simulink model "lab7_block"  (R2017b)
settings: Solver=VariableStepAuto  StartTime=0.0  StopTime=10  MaxStep=0.001  RelTol=1e-3
settings Model: Creator=user  LastModifiedBy=HONOR
settings SolverCC: AutoInsertRateTranBlk=on
settings DataIOCC: LimitDataPoints=on  SaveOutput=off  SignalLogging=off  SaveTime=off
settings OptimizationCC: LifeSpan=inf
settings DebuggingCC: AlgebraicLoopMsg=error  SingleTaskRateTransMsg=error  AllowSymbolicDim=off  SFUnexpectedBacktrackingDiag=warning  SFNoUnconditionalDefaultTransitionDiag=warning  SFExecutionAtInitializationDiag=none
settings CodeAppCC: StateflowObjectComments=on
settings GRTTargetCC: TargetLangStandard=C89/C90 (ANSI)  GeneratePreprocessorConditionals=Disable all
settings ConfigComp: CovMetricSettings=dw  CovHtmlReporting=on  CovSaveCumulativeToWorkspaceVar=on  CovSaveSingleToWorkspaceVar=on  CovExternalEMLEnable=off

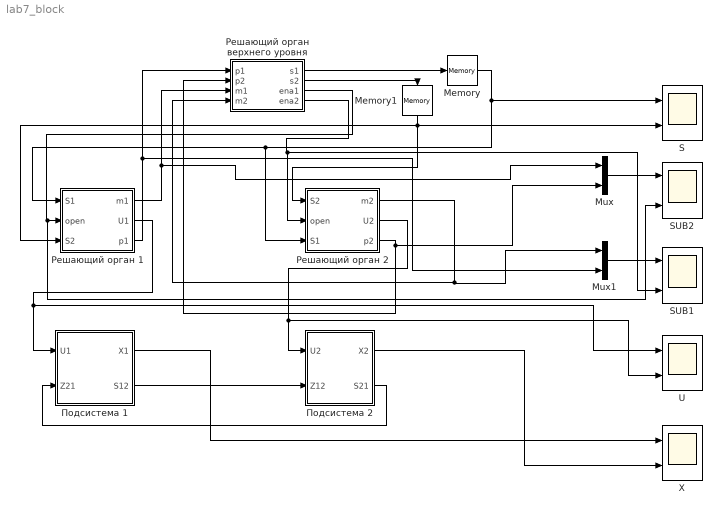
== system lab7_block ==
  Memory : Memory  InitialCondition=0.5
  Memory1 : Memory  InitialCondition=0.5
  Mux : Mux  Inputs=2
  Mux1 : Mux  Inputs=2
  S : Scope  NumInputPorts=2
  SUB1 : Scope  NumInputPorts=2
  SUB2 : Scope  NumInputPorts=2
  U : Scope  NumInputPorts=2
  X : Scope  NumInputPorts=2
  Подсистема 1 : Subsystem
  Подсистема 2 : Subsystem
  Решающий орган 1 : Subsystem
  Решающий орган 2 : Subsystem
  Решающий орган верхнего уровня : MATLAB Function  TreatAsAtomicUnit=on
  wires:
  Подсистема 1/2(S12) -> Подсистема 2/2(Z12)
  Подсистема 2/2(S21) -> Подсистема 1/2(Z21)
  Решающий орган верхнего уровня/1(s1) -> Memory/1
  Решающий орган верхнего уровня/2(s2) -> Memory1/1
  Решающий орган 1/2(U1) -> Подсистема 1/1(U1), U/1
  Решающий орган 2/2(U2) -> U/2, Подсистема 2/1(U2)
  Решающий орган верхнего уровня/3(ena1) -> SUB2/2, Решающий орган 1/2(open)
  Решающий орган верхнего уровня/4(ena2) -> Решающий орган 2/2(open), SUB1/2
  Mux/1 -> SUB2/1
  Mux1/1 -> SUB1/1
  Memory/1 -> S/1, Решающий орган 2/3(S1), Решающий орган 1/1(S1)
  Memory1/1 -> Решающий орган 1/3(S2), Решающий орган 2/1(S2), S/2
  Решающий орган 1/1(m1) -> Mux/1, Решающий орган верхнего уровня/3(m1)
  Решающий орган 1/3(p1) -> Mux1/2, Решающий орган верхнего уровня/1(p1)
  Решающий орган 2/1(m2) -> Mux1/1, Решающий орган верхнего уровня/4(m2)
  Решающий орган 2/3(p2) -> Mux/2, Решающий орган верхнего уровня/2(p2)
  Подсистема 1/1(X1) -> X/1
  Подсистема 2/1(X2) -> X/2

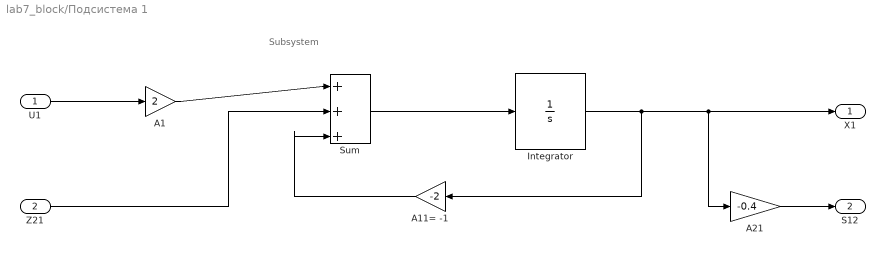
== system lab7_block/Подсистема 1 ==
  note: Subsystem
  U1 : Inport
  Z21 : Inport  Port=2
  A1 : Gain  Gain=2
  A11= -1 : Gain  Gain=-2
  A21 : Gain  Gain=-0.4
  Integrator : Integrator
  Sum : Sum  Inputs=|+++
  X1 : Outport
  S12 : Outport  Port=2
  wires:
  Integrator/1 -> A21/1, X1/1, A11= -1/1
  Sum/1 -> Integrator/1
  Z21/1 -> Sum/2
  A21/1 -> S12/1
  A11= -1/1 -> Sum/3
  A1/1 -> Sum/1
  U1/1 -> A1/1

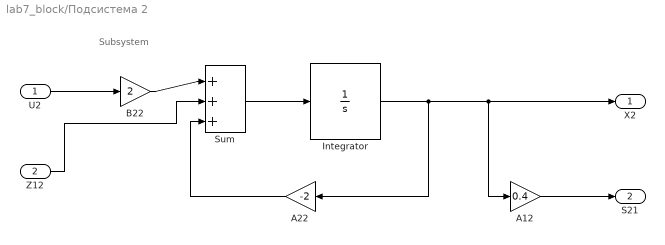
== system lab7_block/Подсистема 2 ==
  note: Subsystem
  U2 : Inport
  Z12 : Inport  Port=2
  A12 : Gain  Gain=0.4
  A22 : Gain  Gain=-2
  B22 : Gain  Gain=2
  Integrator : Integrator
  Sum : Sum  Inputs=|+++
  X2 : Outport
  S21 : Outport  Port=2
  wires:
  A12/1 -> S21/1
  Z12/1 -> Sum/2
  Integrator/1 -> A12/1, X2/1, A22/1
  A22/1 -> Sum/3
  Sum/1 -> Integrator/1
  B22/1 -> Sum/1
  U2/1 -> B22/1

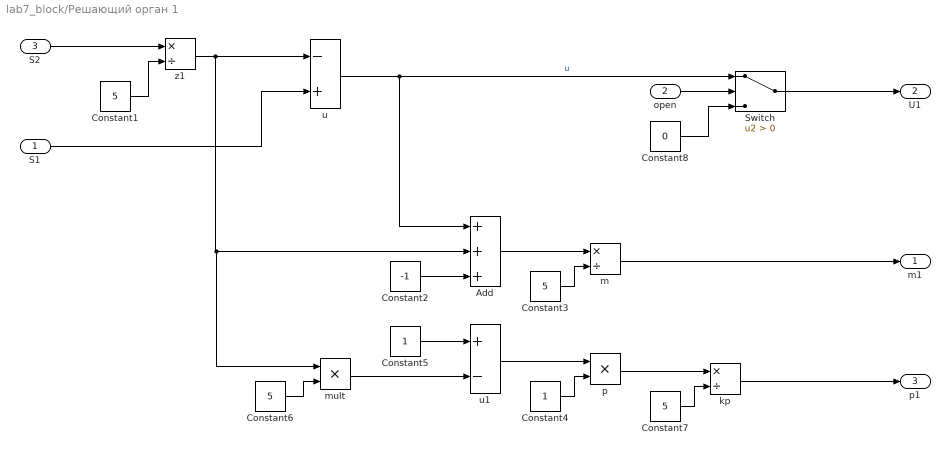
== system lab7_block/Решающий орган 1 ==
  S1 : Inport
  open : Inport  Port=2
  S2 : Inport  Port=3
  Add : Sum  Inputs=+++
  Constant{1,3,6..7} (4 alike) : Constant  Value=5
  Constant2 : Constant  Value=-1
  Constant4 : Constant
  Constant5 : Constant
  Constant8 : Constant  Value=0
  Switch : Switch  Criteria=u2 > Threshold
  kp : Product  Inputs=*/
  m : Product  Inputs=*/
  mult : Product  Inputs=**
  p : Product  Inputs=**
  u : Sum  Inputs=-+
  u1 : Sum  Inputs=+-
  z1 : Product  Inputs=*/
  m1 : Outport
  U1 : Outport  Port=2
  p1 : Outport  Port=3
  wires:
  Switch/1 -> U1/1
  open/1 -> Switch/2
  Constant8/1 -> Switch/3
  Constant1/1 -> z1/2
  S2/1 -> z1/1
  u/1 -> Add/1, Switch/1  "u"
  z1/1 -> mult/1, Add/2, u/1
  S1/1 -> u/2
  Add/1 -> m/1
  Constant2/1 -> Add/3
  Constant3/1 -> m/2
  m/1 -> m1/1
  u1/1 -> p/1
  Constant4/1 -> p/2
  mult/1 -> u1/2
  Constant5/1 -> u1/1
  Constant6/1 -> mult/2
  Constant7/1 -> kp/2
  p/1 -> kp/1
  kp/1 -> p1/1

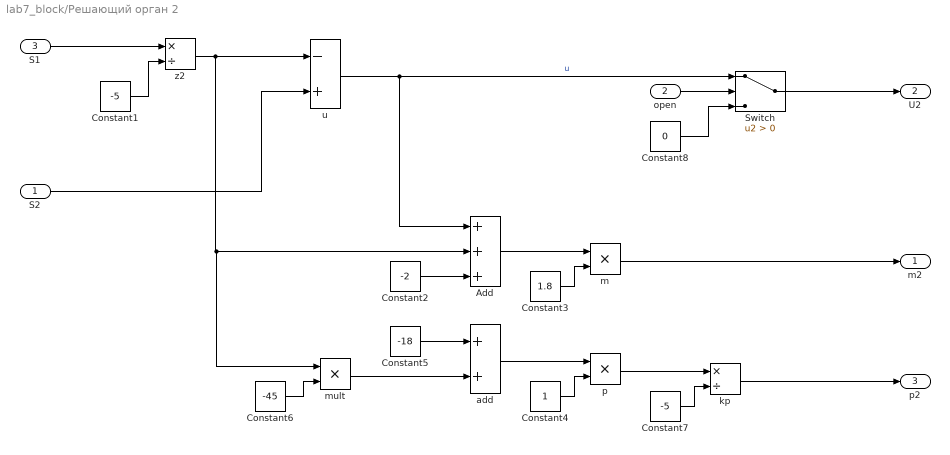
== system lab7_block/Решающий орган 2 ==
  S2 : Inport
  open : Inport  Port=2
  S1 : Inport  Port=3
  Add : Sum  Inputs=+++
  Constant1 : Constant  Value=-5
  Constant2 : Constant  Value=-2
  Constant3 : Constant  Value=1.8
  Constant4 : Constant
  Constant5 : Constant  Value=-18
  Constant6 : Constant  Value=-45
  Constant7 : Constant  Value=-5
  Constant8 : Constant  Value=0
  Switch : Switch  Criteria=u2 > Threshold
  add : Sum
  kp : Product  Inputs=*/
  m : Product  Inputs=**
  mult : Product  Inputs=**
  p : Product  Inputs=**
  u : Sum  Inputs=-+
  z2 : Product  Inputs=*/
  m2 : Outport
  U2 : Outport  Port=2
  p2 : Outport  Port=3
  wires:
  m/1 -> m2/1
  Constant5/1 -> add/1
  Add/1 -> m/1
  Constant6/1 -> mult/2
  S1/1 -> z2/1
  Constant4/1 -> p/2
  Constant2/1 -> Add/3
  Switch/1 -> U2/1
  mult/1 -> add/2
  open/1 -> Switch/2
  Constant1/1 -> z2/2
  z2/1 -> mult/1, Add/2, u/1
  Constant3/1 -> m/2
  u/1 -> Add/1, Switch/1  "u"
  add/1 -> p/1
  S2/1 -> u/2
  Constant8/1 -> Switch/3
  Constant7/1 -> kp/2
  p/1 -> kp/1
  kp/1 -> p2/1

== matlab function lab7_block/Решающий орган верхнего уровня ==
  data: p1 input; s1 output; p2 input; m1 input; m2 input; s2 output; ena1 output; ena2 output
function [s1, s2, ena1, ena2] = fcn(p1, p2, m1, m2)
persistent ds1_t;
persistent ds2_t;
persistent s1_t;
persistent s2_t;
persistent ena1_t;
persistent ena2_t;
eps = 0.0002;  % Величина отклонения оценки от реального значения
step = 0.03;  % Шаг изменения множителей p
% Инициализация
if(isempty(s1_t))
    s1_t = 1.;%-12.5;
    s2_t = 1.;%12.5;
    ds1_t = 0;
    ds2_t = 0;
    ena1_t = 0;
    ena2_t = 0;
    s1 = s1_t;
    s2 = s2_t;
    ena1 = ena1_t;
    ena2 = ena2_t;
    return;
end
if(abs((m1-p2)) > eps || abs((m2-p1)) > eps)
   s1_t = s1_t-step*(m1-p2);%+
   ena1_t = 0;    
   s2_t = s2_t-step*(m2-p1);%-
   ena2_t = 0;
else
   ena1_t = 1;
   ena2_t = 1; 
end
s1 = s1_t;
s2 = s2_t;
ena1 = ena1_t;
ena2 = ena2_t;
end
